simulink model "discrete_p1P_4error_round_additive"  (R2015b)
settings: Solver=VariableStepAuto  StartTime=0.0  StopTime=10.0  RelTol=1e-3
values from neighbouring files (symbols this model uses):
  A = 2    [FYP_MILP_para_setup.m]
  Beta = 0.2    [FYP_MILP_para_setup.m]
  f_e_max = max(x_f_e)    [FYP_set_plant1_para_final_final_fe.m]
  K = 1    [FYP_MILP_para_setup.m]
  k_u = x(2*N+1:3*N)    [FYP_stage1_plant1_3error_round_final_final.m]
  p = 0.5    [FYP_MILP_para_setup.m]
  Ts = 0.01    [FYP_MILP_para_setup.m]
  u_e_max = max(x_u_e)    [FYP_set_plant1_para_final_final_ue.m]
  v_e_max = max(x_v_e)    [FYP_set_plant1_para_final_final_ve.m]
  y_q_max = max(abs(fval_yq))    [FYP_set_plant1_para_final_final_yq.m]
undefined symbols (not defined in the file or in its folder): Gh, he1, l
libraries: simulink x7
settings Model: Creator=bowenpyk  LastModifiedBy=bowenpyk

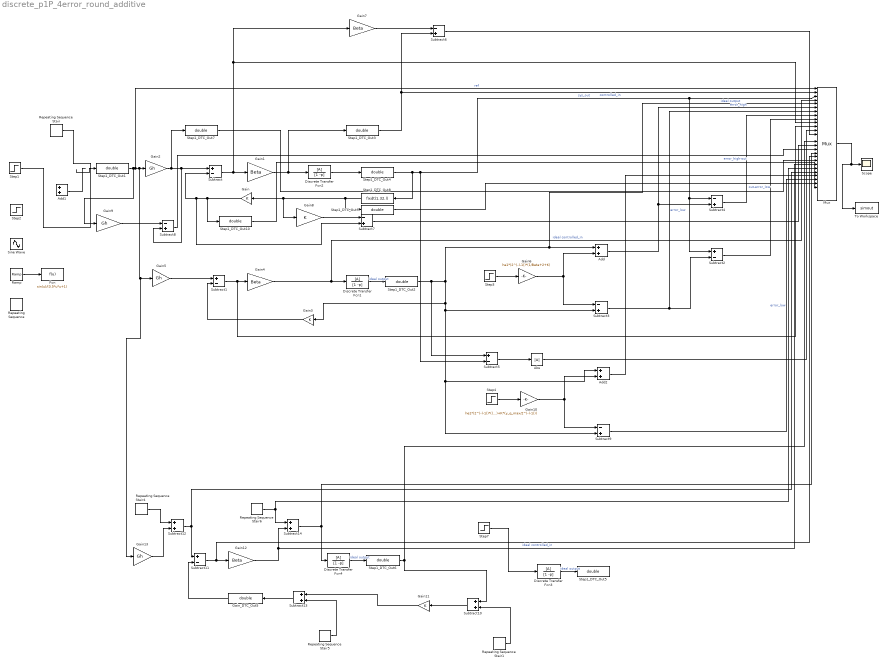
== system discrete_p1P_4error_round_additive ==
  Abs : Abs
  Add : Sum
  Add1 : Sum
  Add2 : Sum
  Discrete Transfer Fcn1 : DiscreteTransferFcn  Numerator=[A]  Denominator=[1 -p]  SampleTime=Ts  RndMeth=Nearest
  Discrete Transfer Fcn2 : DiscreteTransferFcn  Numerator=[A]  Denominator=[1 -p]  SampleTime=Ts  StateDataTypeStr=fixdt(1,32,20)  NumCoefDataTypeStr=fixdt(1,32,20)  DenCoefDataTypeStr=fixdt(1,32,20)  NumProductDataTypeStr=fixdt(1,32,20)  DenProductDataTypeStr=fixdt(1,32,20)  NumAccumDataTypeStr=fixdt(1,32,20)  DenAccumDataTypeStr=fixdt(1,32,20)  OutDataTypeStr=fixdt(1,32,20)  RndMeth=Nearest
  Discrete Transfer Fcn3 : DiscreteTransferFcn  Numerator=[A]  Denominator=[1 -p]  SampleTime=Ts  RndMeth=Nearest
  Discrete Transfer Fcn4 : DiscreteTransferFcn  Numerator=[A]  Denominator=[1 -p]  SampleTime=Ts  RndMeth=Nearest
  Fcn : Fcn  Expr=sin(u)/(0.5*u*u+1)
  Gain : Gain  Gain=K  OutDataTypeStr=fixdt(1,32,l)  RndMeth=Nearest
  Gain1 : Gain  Gain=Beta  OutDataTypeStr=fixdt(1,32,l)  RndMeth=Nearest
  Gain10 : Gain  Gain=he1*(2^(-l-1))*((u_e_max/2^(-l-1))/Beta+(f_e_max/2^(-l-1))+(v_e_max/2^(-l-1))+K*(y_q_max/2^(-l-1)))  OutDataTypeStr=double  RndMeth=Nearest  LockScale=on
  Gain11 : Gain  Gain=K  OutDataTypeStr=double  RndMeth=Nearest
  Gain12 : Gain  Gain=Beta  OutDataTypeStr=double  RndMeth=Nearest
  Gain13 : Gain  Gain=Gh  OutDataTypeStr=double  RndMeth=Nearest
  Gain2 : Gain  Gain=Gh  OutDataTypeStr=fixdt(1,32,l)  RndMeth=Nearest
  Gain3 : Gain  Gain=K  OutDataTypeStr=double  RndMeth=Nearest
  Gain4 : Gain  Gain=Beta  OutDataTypeStr=double  RndMeth=Nearest
  Gain5 : Gain  Gain=Gh  OutDataTypeStr=double  RndMeth=Nearest
  Gain6 : Gain  Gain=he1*(2^(-l-1))*(1/Beta+2+K)  OutDataTypeStr=double  RndMeth=Nearest  LockScale=on
  Gain7 : Gain  Gain=Beta  OutDataTypeStr=double  RndMeth=Nearest
  Gain8 : Gain  Gain=K  OutDataTypeStr=double  RndMeth=Nearest
  Gain9 : Gain  Gain=Gh  OutDataTypeStr=double  RndMeth=Nearest
  Gain_DTC_Out5 : DataTypeConversion  OutDataTypeStr=double  RndMeth=Nearest
  Mux : Mux  Inputs=30
      settings: DisplayOption=signals
  Ramp : simulink/Sources/Ramp  slope=1  start=0  X0=0
  Repeating Sequence : simulink/Sources/Repeating Sequence  rep_seq_t=[0 2]  rep_seq_y=[0 2]
  Repeating Sequence Stair : simulink/Sources/Repeating Sequence Stair  OutValues=r_p1  tsamp=0.01  OutMin=[]  OutMax=[]  OutDataTypeStr=double  OutputDataTypeScalingMode=double  OutDataType=fixdt(0,8)  ConRadixGroup=Best Precision: Vector-wise  OutScaling=2^-12
  Repeating Sequence Stair1 : simulink/Sources/Repeating Sequence Stair  OutValues=y_q1  tsamp=0.01  OutMin=[]  OutMax=[]  OutDataTypeStr=double  OutputDataTypeScalingMode=double  OutDataType=fixdt(0,8)  ConRadixGroup=Best Precision: Vector-wise  OutScaling=2^-12
  Repeating Sequence Stair4 : simulink/Sources/Repeating Sequence Stair  OutValues=v_e1  tsamp=0.01  OutMin=[]  OutMax=[]  OutDataTypeStr=double  OutputDataTypeScalingMode=double  OutDataType=fixdt(0,8)  ConRadixGroup=Best Precision: Vector-wise  OutScaling=2^-12
  Repeating Sequence Stair5 : simulink/Sources/Repeating Sequence Stair  OutValues=f_e1  tsamp=0.01  OutMin=[]  OutMax=[]  OutDataTypeStr=double  OutputDataTypeScalingMode=double  OutDataType=fixdt(0,8)  ConRadixGroup=Best Precision: Vector-wise  OutScaling=2^-12
  Repeating Sequence Stair6 : simulink/Sources/Repeating Sequence Stair  OutValues=u_e1  tsamp=0.01  OutMin=[]  OutMax=[]  OutDataTypeStr=double  OutputDataTypeScalingMode=double  OutDataType=fixdt(0,8)  ConRadixGroup=Best Precision: Vector-wise  OutScaling=2^-12
  Scope : Scope
  Sine Wave : Sin  SampleTime=0
  Step1 : Step  Time=0  After=0.7  SampleTime=0
  Step1_DTC_Out{1..4,6..7,9..10} (8 alike) : DataTypeConversion  OutDataTypeStr=double  RndMeth=Nearest
  Step1_DTC_Out5 : DataTypeConversion  OutDataTypeStr=double
  Step1_DTC_Out8 : DataTypeConversion  OutDataTypeStr=fixdt(1,32,l)  RndMeth=Nearest
  Step2 : Step  Time=1.5  After=-2  SampleTime=0
  Step3 : Step  Time=0  SampleTime=0
  Step4 : Step  Time=0  SampleTime=0
  Step7 : Step  After=k_u*2^(-l)  SampleTime=0
  Subtract : Sum  Inputs=+-  OutDataTypeStr=double  RndMeth=Nearest
  Subtract{1..2,5,11} (4 alike) : Sum  Inputs=+-  OutDataTypeStr=double
  Subtract{10,12..14} (4 alike) : Sum  OutDataTypeStr=double
  Subtract3 : Sum  Inputs=-+  OutDataTypeStr=double
  Subtract4 : Sum  Inputs=-+  OutDataTypeStr=double
  Subtract6 : Sum  Inputs=-+  OutDataTypeStr=double  RndMeth=Nearest
  Subtract7 : Sum  Inputs=-+  OutDataTypeStr=double  RndMeth=Nearest
  Subtract8 : Sum  Inputs=-+  OutDataTypeStr=double  RndMeth=Nearest
  Subtract9 : Sum  Inputs=-+  OutDataTypeStr=double
  To Workspace : ToWorkspace  VariableName=simout  SaveFormat=Timeseries  SampleTime=-1
  wires:
  Discrete Transfer Fcn2/1 -> Step1_DTC_Out4/1
  Mux/1 -> To Workspace/1, Scope/1
  Gain/1 -> Step1_DTC_Out10/1, Subtract7/2, Subtract/2
  Subtract/1 -> Mux/10, Gain7/1, Gain1/1
  Gain1/1 -> Step1_DTC_Out3/1, Discrete Transfer Fcn2/1
  Step1_DTC_Out1/1 -> Gain9/1, Mux/1, Gain13/1, Gain5/1, Gain2/1  "ref"
  Gain2/1 -> Step1_DTC_Out7/1, Subtract8/2, Subtract/1
  Gain3/1 -> Subtract1/2
  Subtract1/1 -> Gain4/1, Mux/11
  Gain4/1 -> Discrete Transfer Fcn1/1, Mux/4  "ideal controlled_in"
  Gain5/1 -> Subtract1/1
  Step3/1 -> Gain6/1
  Gain6/1 -> Add/2, Subtract3/1
  Add/1 -> Mux/6, Subtract4/2  "error_high"
  Subtract3/1 -> Mux/7, Subtract2/2  "error_low"
  Step1_DTC_Out3/1 -> Mux/2, Subtract6/2  "controlled_in"
  Step1_DTC_Out4/1 -> Step1_DTC_Out8/1, Subtract5/2, Subtract4/1, Subtract2/1, Mux/3  "sys_out"
  Subtract2/1 -> Mux/9  "out-error_low"
  Subtract4/1 -> Mux/8  "error_high-out"
  Step1/1 -> ?
  Add1/1 -> ?
  Ramp/1 -> Fcn/1
  Subtract5/1 -> Abs/1
  Abs/1 -> Mux/12
  Repeating Sequence Stair/1 -> Step1_DTC_Out1/1
  Gain7/1 -> Subtract6/1
  Subtract6/1 -> Mux/13
  Discrete Transfer Fcn1/1 -> Step1_DTC_Out2/1  "ideal output"
  Step7/1 -> Discrete Transfer Fcn3/1
  Discrete Transfer Fcn3/1 -> Step1_DTC_Out5/1  "ideal output"
  Gain11/1 -> Subtract13/1
  Gain_DTC_Out5/1 -> Subtract11/2
  Subtract11/1 -> Mux/19, Gain12/1
  Gain12/1 -> Mux/21, Subtract14/2  "ideal controlled_in"
  Gain13/1 -> Subtract12/2
  Discrete Transfer Fcn4/1 -> Step1_DTC_Out6/1  "ideal output"
  Subtract12/1 -> Mux/23, Subtract11/1
  Repeating Sequence Stair4/1 -> Subtract12/1
  Repeating Sequence Stair5/1 -> Subtract13/2
  Subtract13/1 -> Gain_DTC_Out5/1
  Repeating Sequence Stair6/1 -> Mux/22, Subtract14/1
  Subtract14/1 -> Mux/18, Discrete Transfer Fcn4/1
  Step1_DTC_Out6/1 -> Subtract10/1, Mux/15
  Gain8/1 -> Subtract7/1
  Subtract7/1 -> Mux/16
  Gain9/1 -> Subtract8/1
  Subtract8/1 -> Mux/17
  Step1_DTC_Out7/1 -> Mux/20
  Step1_DTC_Out2/1 -> Subtract5/1, Add2/1, Subtract9/2, Subtract3/2, Gain3/1, Mux/5, Add/1  "ideal output"
  Step4/1 -> Gain10/1
  Gain10/1 -> Add2/2, Subtract9/1
  Subtract9/1 -> Mux/25  "error_low"
  Add2/1 -> Mux/24
  Repeating Sequence Stair1/1 -> Subtract10/2
  Subtract10/1 -> Gain11/1
  Step1_DTC_Out8/1 -> Step1_DTC_Out9/1, Gain8/1, Gain/1
  Step1_DTC_Out9/1 -> Mux/26
  Step1_DTC_Out10/1 -> Mux/27
